simulink model "lookuptable2D"  (Simulink 7.9)
settings: Solver=FixedStepDiscrete  StartTime=0.0  StopTime=10.0  FixedStep=1  RelTol=1e-3
settings Model: Creator=hnine  LastModifiedBy=hnine

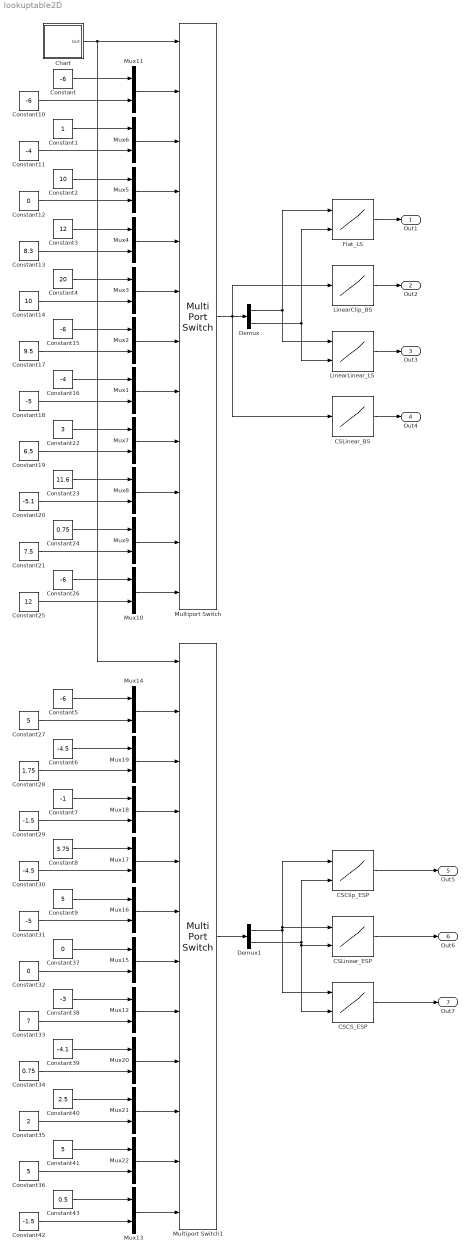
== system lookuptable2D ==
  CSCS_ESP : Lookup_n-D  BreakpointsForDimension1=[ -4 -3 -2 -1 0 1 2 3 4 5 ]  BreakpointsForDimension2=[ -4.5 -3.5 -2.5 -1.5 -0.5 0.5 1.5 2.5 3.5 4.5 ]  IndexSearchMethod=Evenly spaced points  Table="[ 10  1  9  2  8  3  7  4  6  5 ; 12  0 10  2 11  4  9  5  7  4 ; 9 -2  7 16  4  8 20 18  4 -1 ; 6  3 11 -4  8 -6 15  2  1  0 ; 14  2  6 -5 15 16 17  5 -4  8 ; -2 15  2 12  8  3 -1  2 -9 19 ; 15  4  7 16  3  3  2 15 13 -6 ;  5  6  4  7  3  8  2  9  1 10 ; -9 -8 -7 -6 -5 -4 -3 -2 -1  0 ;  4  9  1 -1 -4  9  1  8  2 11  ]"  InterpMethod=Cubic spline  ExtrapMethod=Cubic spline  RndMeth=Simplest  InputSameDT=on
  CSClip_ESP : Lookup_n-D  BreakpointsForDimension1=[ -4 -3 -2 -1 0 1 2 3 4 5 ]  BreakpointsForDimension2=[ -4.5 -3.5 -2.5 -1.5 -0.5 0.5 1.5 2.5 3.5 4.5 ]  IndexSearchMethod=Evenly spaced points  Table="[ 10  1  9  2  8  3  7  4  6  5 ; 12  0 10  2 11  4  9  5  7  4 ; 9 -2  7 16  4  8 20 18  4 -1 ; 6  3 11 -4  8 -6 15  2  1  0 ; 14  2  6 -5 15 16 17  5 -4  8 ; -2 15  2 12  8  3 -1  2 -9 19 ; 15  4  7 16  3  3  2 15 13 -6 ;  5  6  4  7  3  8  2  9  1 10 ; -9 -8 -7 -6 -5 -4 -3 -2 -1  0 ;  4  9  1 -1 -4  9  1  8  2 11  ]"  InterpMethod=Cubic spline  ExtrapMethod=Clip  RndMeth=Simplest  InputSameDT=on
  CSLinear_BS : Lookup_n-D  BreakpointsForDimension1=[ -4 -2 -0.5 .75 3 8 10 11 11.5 15 ]  BreakpointsForDimension2=[ -5 -3 -2.5 0 3 5 6 6.2 7 9 ]  UseOneInputPortForAllInputData=on  Table="[ 10  1  9  2  8  3  7  4  6  5 ; 12  0 10  2 11  4  9  5  7  4 ; 9 -2  7 16  4  8 20 18  4 -1 ; 6  3 11 -4  8 -6 15  2  1  0 ; 14  2  6 -5 15 16 17  5 -4  8 ; -2 15  2 12  8  3 -1  2 -9 19 ; 15  4  7 16  3  3  2 15 13 -6 ;  5  6  4  7  3  8  2  9  1 10 ; -9 -8 -7 -6 -5 -4 -3 -2 -1  0 ;  4  9  1 -1 -4  9  1  8  2 11  ]"  InterpMethod=Cubic spline  RndMeth=Simplest  InputSameDT=on
  CSLinear_ESP : Lookup_n-D  BreakpointsForDimension1=[ -4 -3 -2 -1 0 1 2 3 4 5 ]  BreakpointsForDimension2=[ -4.5 -3.5 -2.5 -1.5 -0.5 0.5 1.5 2.5 3.5 4.5 ]  IndexSearchMethod=Linear search  Table="[ 10  1  9  2  8  3  7  4  6  5 ; 12  0 10  2 11  4  9  5  7  4 ; 9 -2  7 16  4  8 20 18  4 -1 ; 6  3 11 -4  8 -6 15  2  1  0 ; 14  2  6 -5 15 16 17  5 -4  8 ; -2 15  2 12  8  3 -1  2 -9 19 ; 15  4  7 16  3  3  2 15 13 -6 ;  5  6  4  7  3  8  2  9  1 10 ; -9 -8 -7 -6 -5 -4 -3 -2 -1  0 ;  4  9  1 -1 -4  9  1  8  2 11  ]"  InterpMethod=Cubic spline  RndMeth=Simplest  InputSameDT=on
  Chart : Stateflow chart  TreatAsAtomicUnit=on
  Constant{,5,10,15,26} (5 alike) : Constant  Value=-6
  Constant1 : Constant
  Constant11 : Constant  Value=-4
  Constant12 : Constant  Value=0
  Constant13 : Constant  Value=8.3
  Constant14 : Constant  Value=10
  Constant16 : Constant  Value=-4
  Constant17 : Constant  Value=9.5
  Constant18 : Constant  Value=-5
  Constant19 : Constant  Value=6.5
  Constant2 : Constant  Value=10
  Constant20 : Constant  Value=-5.1
  Constant21 : Constant  Value=7.5
  Constant22 : Constant  Value=3
  Constant23 : Constant  Value=11.6
  Constant24 : Constant  Value=0.75
  Constant25 : Constant  Value=12
  Constant{9,27,36,41} (4 alike) : Constant  Value=5
  Constant28 : Constant  Value=1.75
  Constant29 : Constant  Value=-1.5
  Constant3 : Constant  Value=12
  Constant30 : Constant  Value=-4.5
  Constant31 : Constant  Value=-5
  Constant32 : Constant  Value=0
  Constant33 : Constant  Value=7
  Constant34 : Constant  Value=0.75
  Constant35 : Constant  Value=2
  Constant37 : Constant  Value=0
  Constant38 : Constant  Value=-3
  Constant39 : Constant  Value=-4.1
  Constant4 : Constant  Value=20
  Constant40 : Constant  Value=2.5
  Constant42 : Constant  Value=-1.5
  Constant43 : Constant  Value=0.5
  Constant6 : Constant  Value=-4.5
  Constant7 : Constant  Value=-1
  Constant8 : Constant  Value=3.75
  Demux : Demux  Outputs=2
  Demux1 : Demux  Outputs=2
  Flat_LS : Lookup_n-D  BreakpointsForDimension1=[ -4 -2 -0.5 .75 3 8 10 11 11.5 15 ]  BreakpointsForDimension2=[ -5 -3 -2.5 0 3 5 6 6.2 7 9 ]  IndexSearchMethod=Linear search  Table="[ 10  1  9  2  8  3  7  4  6  5 ; 12  0 10  2 11  4  9  5  7  4 ; 9 -2  7 16  4  8 20 18  4 -1 ; 6  3 11 -4  8 -6 15  2  1  0 ; 14  2  6 -5 15 16 17  5 -4  8 ; -2 15  2 12  8  3 -1  2 -9 19 ; 15  4  7 16  3  3  2 15 13 -6 ;  5  6  4  7  3  8  2  9  1 10 ; -9 -8 -7 -6 -5 -4 -3 -2 -1  0 ;  4  9  1 -1 -4  9  1  8  2 11  ]"  InterpMethod=Flat  RndMeth=Simplest  InputSameDT=on
  LinearClip_BS : Lookup_n-D  BreakpointsForDimension1=[ -4 -2 -0.5 .75 3 8 10 11 11.5 15 ]  BreakpointsForDimension2=[ -5 -3 -2.5 0 3 5 6 6.2 7 9 ]  UseOneInputPortForAllInputData=on  Table="[ 10  1  9  2  8  3  7  4  6  5 ; 12  0 10  2 11  4  9  5  7  4 ; 9 -2  7 16  4  8 20 18  4 -1 ; 6  3 11 -4  8 -6 15  2  1  0 ; 14  2  6 -5 15 16 17  5 -4  8 ; -2 15  2 12  8  3 -1  2 -9 19 ; 15  4  7 16  3  3  2 15 13 -6 ;  5  6  4  7  3  8  2  9  1 10 ; -9 -8 -7 -6 -5 -4 -3 -2 -1  0 ;  4  9  1 -1 -4  9  1  8  2 11  ]"  ExtrapMethod=Clip  RndMeth=Simplest  InputSameDT=on
  LinearLinear_LS : Lookup_n-D  BreakpointsForDimension1=[ -4 -2 -0.5 .75 3 8 10 11 11.5 15 ]  BreakpointsForDimension2=[ -5 -3 -2.5 0 3 5 6 6.2 7 9 ]  IndexSearchMethod=Linear search  Table="[ 10  1  9  2  8  3  7  4  6  5 ; 12  0 10  2 11  4  9  5  7  4 ; 9 -2  7 16  4  8 20 18  4 -1 ; 6  3 11 -4  8 -6 15  2  1  0 ; 14  2  6 -5 15 16 17  5 -4  8 ; -2 15  2 12  8  3 -1  2 -9 19 ; 15  4  7 16  3  3  2 15 13 -6 ;  5  6  4  7  3  8  2  9  1 10 ; -9 -8 -7 -6 -5 -4 -3 -2 -1  0 ;  4  9  1 -1 -4  9  1  8  2 11  ]"  RndMeth=Simplest  InputSameDT=on
  Multiport Switch : MultiPortSwitch  DataPortOrder=Zero-based contiguous  Inputs=11  DiagnosticForDefault=None  zeroidx=on
  Multiport Switch1 : MultiPortSwitch  DataPortOrder=Zero-based contiguous  Inputs=11  DiagnosticForDefault=None  zeroidx=on
  Mux{1..22} (22 alike) : Mux  Inputs=2
  Out1 : Outport
  Out2 : Outport  Port=2
  Out3 : Outport  Port=3
  Out4 : Outport  Port=4
  Out5 : Outport  Port=5
  Out6 : Outport  Port=6
  Out7 : Outport  Port=7
  wires:
  Flat_LS/1 -> Out1/1
  Chart/1(out) -> Multiport Switch/1, Multiport Switch1/1
  Constant/1 -> Mux11/1
  Constant1/1 -> Mux6/1
  Constant2/1 -> Mux5/1
  Constant3/1 -> Mux4/1
  Constant4/1 -> Mux3/1
  LinearClip_BS/1 -> Out2/1
  LinearLinear_LS/1 -> Out3/1
  CSClip_ESP/1 -> Out5/1
  CSLinear_BS/1 -> Out4/1
  CSCS_ESP/1 -> Out7/1
  CSLinear_ESP/1 -> Out6/1
  Mux11/1 -> Multiport Switch/2
  Mux6/1 -> Multiport Switch/3
  Mux5/1 -> Multiport Switch/4
  Mux4/1 -> Multiport Switch/5
  Mux3/1 -> Multiport Switch/6
  Mux2/1 -> Multiport Switch/7
  Mux1/1 -> Multiport Switch/8
  Mux7/1 -> Multiport Switch/9
  Mux8/1 -> Multiport Switch/10
  Mux9/1 -> Multiport Switch/11
  Mux10/1 -> Multiport Switch/12
  Multiport Switch/1 -> Demux/1, LinearClip_BS/1, CSLinear_BS/1
  Demux/1 -> Flat_LS/1, LinearLinear_LS/1
  Demux/2 -> Flat_LS/2, LinearLinear_LS/2
  Constant10/1 -> Mux11/2
  Constant11/1 -> Mux6/2
  Constant12/1 -> Mux5/2
  Constant13/1 -> Mux4/2
  Constant14/1 -> Mux3/2
  Constant15/1 -> Mux2/1
  Constant16/1 -> Mux1/1
  Constant22/1 -> Mux7/1
  Constant23/1 -> Mux8/1
  Constant24/1 -> Mux9/1
  Constant17/1 -> Mux2/2
  Constant18/1 -> Mux1/2
  Constant19/1 -> Mux7/2
  Constant20/1 -> Mux8/2
  Constant21/1 -> Mux9/2
  Constant26/1 -> Mux10/1
  Constant25/1 -> Mux10/2
  Mux14/1 -> Multiport Switch1/2
  Mux19/1 -> Multiport Switch1/3
  Mux18/1 -> Multiport Switch1/4
  Mux17/1 -> Multiport Switch1/5
  Mux16/1 -> Multiport Switch1/6
  Mux15/1 -> Multiport Switch1/7
  Mux12/1 -> Multiport Switch1/8
  Mux20/1 -> Multiport Switch1/9
  Mux21/1 -> Multiport Switch1/10
  Mux22/1 -> Multiport Switch1/11
  Mux13/1 -> Multiport Switch1/12
  Multiport Switch1/1 -> Demux1/1
  Demux1/1 -> CSClip_ESP/1, CSLinear_ESP/1, CSCS_ESP/1
  Demux1/2 -> CSClip_ESP/2, CSLinear_ESP/2, CSCS_ESP/2
  Constant5/1 -> Mux14/1
  Constant6/1 -> Mux19/1
  Constant7/1 -> Mux18/1
  Constant8/1 -> Mux17/1
  Constant9/1 -> Mux16/1
  Constant27/1 -> Mux14/2
  Constant28/1 -> Mux19/2
  Constant29/1 -> Mux18/2
  Constant30/1 -> Mux17/2
  Constant31/1 -> Mux16/2
  Constant37/1 -> Mux15/1
  Constant38/1 -> Mux12/1
  Constant39/1 -> Mux20/1
  Constant40/1 -> Mux21/1
  Constant41/1 -> Mux22/1
  Constant32/1 -> Mux15/2
  Constant33/1 -> Mux12/2
  Constant34/1 -> Mux20/2
  Constant35/1 -> Mux21/2
  Constant36/1 -> Mux22/2
  Constant42/1 -> Mux13/2
  Constant43/1 -> Mux13/1

== stateflow chart Chart ==
  state count
    en: out = 0;
    du: out = out + 1;
  (default) -> count
  count -> count : [ out >= 10 ]
  data: out output double =0
